simulink model "Practica2p1"  (R2015a)
settings: Solver=ode45  StartTime=0.0  StopTime=100.0  MaxStep=0.1  RelTol=1e-3
settings Model: CovSFcnEnable=off  Creator=usuario_local  LastModifiedBy=Jota
settings DebuggingCC: SolverPrmCheckMsg=warning

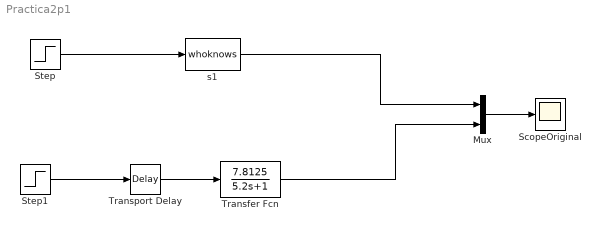
== system Practica2p1 ==
  Mux : Mux  Inputs=2
  "ScopeOriginal " : Scope
      settings: SaveName=ScopeDataPlantaOriginal
  Step : Step  SampleTime=0
  Step1 : Step  SampleTime=0
  Transfer Fcn : TransferFcn  Numerator=[7.8125]  Denominator=[5.2 1]
  Transport Delay : TransportDelay  DelayTime=3.6
  s1 : M-S-Function  FunctionName=whoknows  Parameters=L, P1, P2, T, R  mask{L=8, P1=1, P2=7, T=1, R=0}
      mask prompts: L "Laboratorio"; P1 "Primer digito del Puesto"; P2 "Segundo digito del Puesto"; T "Tipo de Planta"; R "Ruido"
      mask Display: disp('Sistema')
  wires:
  Step/1 -> s1/1
  s1/1 -> Mux/1
  Transport Delay/1 -> Transfer Fcn/1
  Step1/1 -> Transport Delay/1
  Transfer Fcn/1 -> Mux/2
  Mux/1 -> "ScopeOriginal "/1
